simulink model "SF007A_SysFricLrng"  (R2013b)
settings: Solver=FixedStepDiscrete  SolverMode=SingleTasking  StartTime=0.0  StopTime=1  FixedStep=0.002  RelTol=1e-3
PostLoadFcn:
  | , if any(exist('dsrtsu_mdlpostloadfcn', 'file') == [2, 3, 6]), try dsrtsu_mdlpostloadfcn('Execute', bdroot); catch fprintf('Error in PostLoadFcn (dsrtsu_mdlpostloadfcn) for model "%s":\n %s\n', bdroot, lasterr); end, end,
undefined symbols (not defined in the file): ARCHGLBPRM_100MILLISEC_SEC_F32, ARCHGLBPRM_10MILLISEC_SEC_F32, ARCHGLBPRM_180OVERPI_ULS_F32, CONV100MICROSECTOSEC_ULS_F32, FLTINJ_SYSFRICLRNG_SYSFRICOFFS, FricLrngData, HiFricNtc, HWPTNUM_CNT_U08, HWPTNUMSUB1_CNT_U08, HWVELDECDIR_ULS_U08, HWVELINCDIR_ULS_U08, IDXCALCNSCAGFAC_ULS_U08, IDXSELN1_ULS_U08, IDXSELN2_ULS_U08, IDXSELN3_ULS_U08, LRNGENASCAFAC_MILLISEC_U32, NtcSts1, SCAGFACQUARTER_CNT_F32, SCAGFACTEN_CNT_U16, SECIDXSELN_ULS_U08, SysFricLrngBasLineEolFric, SysFricLrngBasLineFric, SysFricLrngBasLineHys, SysFricLrngBasLineRngCntr, SysFricLrngEolFricDifScagFac, SysFricLrngFricChgWght, SysFricLrngFricDiagcThd, SysFricLrngFricDiagcTiThd, SysFricLrngFricHysHwAgPt, SysFricLrngGain, SysFricLrngHwPosnAuthyThd, SysFricLrngHwVelConstrLim, SysFricLrngHwVelHiLim, SysFricLrngHwVelLoLim, SysFricLrngIgnCycFricChgLim, SysFricLrngLatAHiLim, SysFricLrngLatALoLim, SysFricLrngMaskVehSpd, SysFricLrngOperMod1, SysFricLrngRngCntrThd, SysFricLrngThd, SysFricLrngTHiLim, SysFricLrngTLoLim, SysFricLrngVehSpd, SYSFRICOFFSLIM_HWNWTMTR_F32, VEHSPDPTNUM1_ULS_U08, VEHSPDPTNUM2_ULS_U08
libraries: Fil x19, simulink x17, NxtrLim x10, NxtrAbslt x3, NxtrNvM x2, FixdToFloat x2, FloatToFixd x1, LnrIntrpn x1
(part 4 of 7)

== system SF007A_SysFricLrng/SysFricLrng/SysFricLrngPer1/RunningAndCalibrationModes/FricLearning/Gate Calculation ==
  SelHwAg : Inport
  IC : Inport  Port=2
  Add1 : Sum
  Constant2 : Constant  Value=HWPTNUMSUB1_CNT_U08
  Constant3 : Constant  Value=SysFricLrngFricHysHwAgPt
  Constant4 : Constant  OutDataTypeStr=uint8
      settings: AttributesFormatString=%<OutDataTypeStr>
  CopyRight2 : Subsystem  Description=|  mask(Copyright Information){none=on}
      | Copyright info block.                                               
      |                                                                     
      | Place copyright information at the top of every subsystem in design.
      mask prompts: none "No parameters"
      mask help: Place copyright information at the top of every subsystem in design.
      mask Display:
      | NxtrConf = 'Nexteer Confidential';
      | 
      | sys = bdroot; %handle for the current model ("system")
      | first = get_param(sys,'Created');
      | first = first(end-3:end);  %year is last four digits
      | 
      | last = get_param(sys,'LastModifiedDate');
      | if isempty(last)
      |     last = datestr(now,'yyyy');
      | else
      |     last = last(end-3:end);
      | end
      | 
      | if strcmp(first,last)
      |     fprintf('%s -- Copyright %s Nexteer',NxtrConf,first)
      | else
      |     fprintf('%s -- %s%s- %s Nexteer',NxtrConf,char(169),first,last)
      | end
  Logical Operator : Logic  AllPortsSameDT=off  OutDataTypeStr=boolean
  Logical Operator1 : Logic  Operator=OR  AllPortsSameDT=off  OutDataTypeStr=boolean
  Relational Operator : RelationalOperator  Operator=<  OutDataTypeStr=boolean
  Relational Operator1 : RelationalOperator  Operator=<  OutDataTypeStr=boolean
  Relational Operator2 : RelationalOperator  OutDataTypeStr=boolean
  Selector : Selector  IndexOptions=Index vector (port)  Indices=[1 3]  OutputSizes=1
  Selector1 : Selector  IndexOptions=Index vector (port)  Indices=[1 3]  OutputSizes=1
  While Iterator : WhileIterator  MaxIters=-1  ShowIterationPort=on
  Gate : Outport
  wires:
  IC/1 -> While Iterator/2
  Constant3/1 -> Selector/1, Selector1/1
  Constant2/1 -> Relational Operator/2
  Relational Operator/1 -> Logical Operator/1
  Add1/1 -> Selector1/2
  Constant4/1 -> Add1/2
  Logical Operator1/1 -> Logical Operator/2
  Logical Operator/1 -> While Iterator/1
  SelHwAg/1 -> [SelHwAg]
  [SelHwAg] -> Relational Operator1/1
  Selector/1 -> Relational Operator1/2
  Relational Operator1/1 -> Logical Operator1/1
  Selector1/1 -> Relational Operator2/2
  [SelHwAg] -> Relational Operator2/1
  Relational Operator2/1 -> Logical Operator1/2
  While Iterator/1 -> Gate/1, Relational Operator/1, Selector/2, Add1/1

== system SF007A_SysFricLrng/SysFricLrng/SysFricLrngPer1/RunningAndCalibrationModes/FricLearning/Indices Calculation ==
  note: Code: (Zero Based Index)                       ||   Model (One Based Index)
      | -----------------------------------------------------||----------------------------------------------------
      | VSIdx | OffsInc | OffsDec|Offs(0)|Offs(1) ||VSIdx | OffsInc | OffsDec|Offs(0)|Offs(1)
      | -----------------------------------------------------------------------------------------------------------
      |      0    |    0      |  1          |  0       |    1      ||   1      |   1         |  2         | 1      |   2
      |      1    |    2      |  3          |  2       |    3      ||   2      |   3         |  4         | 3      |   4
      |      2    |    4      |  5          |  4       |    5      ||   3      |   5         |  6         | 5      |   6
      |      3    |    6      |  7          |  6       |    7      ||   4      |   7         |  8         | 7      |   8
  note: Note: Mapping of values between Zero Based and one based Index
  HwVelDir : Inport
  VehSpdIdx : Inport  Port=2
  Add1 : Sum  Inputs=+-
  Add2 : Sum
  Add3 : Sum  Inputs=+-
  Constant1 : Constant  OutDataTypeStr=uint8
      settings: AttributesFormatString=%<OutDataTypeStr>
  Constant2 : Constant  Value=IDXCALCNSCAGFAC_ULS_U08
  Constant3 : Constant  OutDataTypeStr=uint8
      settings: AttributesFormatString=%<OutDataTypeStr>
  CopyRight2 : Subsystem  Description=|  mask(Copyright Information){none=on}
      | Copyright info block.                                               
      |                                                                     
      | Place copyright information at the top of every subsystem in design.
      mask prompts: none "No parameters"
      mask help: Place copyright information at the top of every subsystem in design.
      mask Display:
      | NxtrConf = 'Nexteer Confidential';
      | 
      | sys = bdroot; %handle for the current model ("system")
      | first = get_param(sys,'Created');
      | first = first(end-3:end);  %year is last four digits
      | 
      | last = get_param(sys,'LastModifiedDate');
      | if isempty(last)
      |     last = datestr(now,'yyyy');
      | else
      |     last = last(end-3:end);
      | end
      | 
      | if strcmp(first,last)
      |     fprintf('%s -- Copyright %s Nexteer',NxtrConf,first)
      | else
      |     fprintf('%s -- %s%s- %s Nexteer',NxtrConf,char(169),first,last)
      | end
  Product : Product
  DeltaIdxOffsInc : Outport
  DeltaIdxOffs : Outport  Port=2
  DeltaIdxOffsDec : Outport  Port=3
  wires:
  Product/1 -> DeltaIdxOffsDec/1, Add3/1, Add2/2
  HwVelDir/1 -> Add2/1
  Constant2/1 -> Product/2
  VehSpdIdx/1 -> Product/1
  Add3/1 -> DeltaIdxOffsInc/1
  Constant3/1 -> Add3/2
  Add2/1 -> Add1/1
  Add1/1 -> DeltaIdxOffs/1
  Constant1/1 -> Add1/2

== stateflow chart SF007A_SysFricLrng/SysFricLrng/SysFricLrngPer1/RunningAndCalibrationModes/FricLearning/Calculate Average Friction/NTC PASS /SetNtcSts/SetNtcSts/ISO Fault Debounce Design ==
  note: NTCSTS_PASSD           (0)
      | NTCSTS_FAILD             (1)
      | NTCSTS_PREPASSD   (2)
      | NTCSTS_PREFAILD     (3)
      |
      | SIGQLFR_NORES        (0)
      | SIGQLFR_PASSD         (1)
      | SIGQLFR_FAILD           (2)
  note: Pass Loop
  note: Fail Loop
  note: 
  (default) -> (junction 89)
  (junction 89) -> (junction 95) [order 1] : [NtcSts ==3]
  (junction 89) -> (junction 93) [order 2] : [NtcSts ==2]
  (junction 89) -> (junction 141) [order 3] : [NtcSts ==1]
      | { ErrAcc = 32767;
      | Qualifier =2;
      |  }
  (junction 89) -> (junction 141) [order 4] : [NtcSts ==0]
      | { ErrAcc = -32768;
      | Qualifier=1;
      | }
  (junction 95) -> (junction 103) [order 2]
  (junction 95) -> (junction 111) [order 1] : [ErrAcc <=0]
      | {ErrAcc = DebStep;}
  (junction 93) -> (junction 123) [order 2] : {
      | ErrAcc = ErrAcc - DebStep;
      | }
  (junction 93) -> (junction 123) [order 1] : [(ErrAcc - DebStep) <= -32768]
      | { ErrAcc = -32768;
      | Qualifier=1;
      | }
  (junction 103) -> (junction 111) [order 1] : [(ErrAcc + DebStep) <32767]
      | {ErrAcc = ErrAcc + DebStep;}
  (junction 103) -> (junction 111) [order 2] : {ErrAcc = 32767;
      | Qualifier =2;}
  (junction 123) -> (junction 141)
  (junction 111) -> (junction 141)
  (junction 141) -> (junction 159) [order 2] : {ErrAcc = 0;
      | Qualifier =0;
      | }
  (junction 141) -> (junction 159) [order 1] : [SvcClr ==0]
  data: NtcSts input Enum: NtcSts1; Qualifier output uint8; DebStep input uint16; ErrAcc local single; SvcClr input

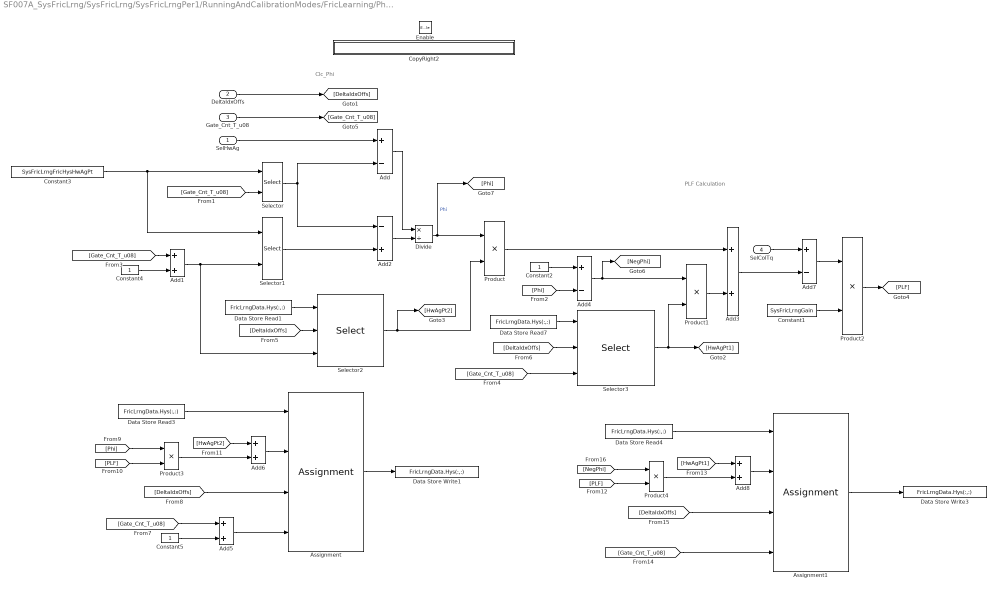
== system SF007A_SysFricLrng/SysFricLrng/SysFricLrngPer1/RunningAndCalibrationModes/FricLearning/Phi Calculation ==
  note: Clc_Phi
  note: PLF Calculation
  SelHwAg : Inport
  DeltaIdxOffs : Inport  Port=2
  Gate_Cnt_T_u08 : Inport  Port=3
  SelColTq : Inport  Port=4
  Enable : EnablePort
  Add : Sum  Inputs=+-
  Add{1,3,5..6,8} (5 alike) : Sum
  Add2 : Sum  Inputs=-+
  Add4 : Sum  Inputs=+-
  Add7 : Sum  Inputs=+-
  Assignment : Assignment  NumberOfDimensions=2  IndexOptions=Index vector (port),Index vector (port)  Indices=1,1  OutputSizes=1,1
  Assignment1 : Assignment  NumberOfDimensions=2  IndexOptions=Index vector (port),Index vector (port)  Indices=1,1  OutputSizes=1,1
  Constant1 : Constant  Value=SysFricLrngGain
  Constant2 : Constant  OutDataTypeStr=single
      settings: AttributesFormatString=%<OutDataTypeStr>
  Constant3 : Constant  Value=SysFricLrngFricHysHwAgPt
  Constant4 : Constant  OutDataTypeStr=uint16
      settings: AttributesFormatString=%<OutDataTypeStr>
  Constant5 : Constant  OutDataTypeStr=uint16
      settings: AttributesFormatString=%<OutDataTypeStr>
  CopyRight2 : Subsystem  Description=|  mask(Copyright Information){none=on}
      | Copyright info block.                                               
      |                                                                     
      | Place copyright information at the top of every subsystem in design.
      mask prompts: none "No parameters"
      mask help: Place copyright information at the top of every subsystem in design.
      mask Display:
      | NxtrConf = 'Nexteer Confidential';
      | 
      | sys = bdroot; %handle for the current model ("system")
      | first = get_param(sys,'Created');
      | first = first(end-3:end);  %year is last four digits
      | 
      | last = get_param(sys,'LastModifiedDate');
      | if isempty(last)
      |     last = datestr(now,'yyyy');
      | else
      |     last = last(end-3:end);
      | end
      | 
      | if strcmp(first,last)
      |     fprintf('%s -- Copyright %s Nexteer',NxtrConf,first)
      | else
      |     fprintf('%s -- %s%s- %s Nexteer',NxtrConf,char(169),first,last)
      | end
  Data Store Read{1,3..4,7} (4 alike) : DataStoreRead  Priority=1  DataStoreName=FricLrngData  DataStoreElements=FricLrngData.Hys(:,:)
      settings: AttributesFormatString=Priority: %<Priority>
  Data Store Write1 : DataStoreWrite  Priority=2  DataStoreName=FricLrngData  DataStoreElements=FricLrngData.Hys(:,:)
      settings: AttributesFormatString=Priority: %<Priority>
  Data Store Write3 : DataStoreWrite  Priority=2  DataStoreName=FricLrngData  DataStoreElements=FricLrngData.Hys(:,:)
      settings: AttributesFormatString=Priority: %<Priority>
  Divide : Product  Inputs=*/
  Product{,1..4} (5 alike) : Product
  Selector : Selector  IndexOptions=Index vector (port)  Indices=[1 3]  OutputSizes=1
  Selector1 : Selector  IndexOptions=Index vector (port)  Indices=[1 3]  OutputSizes=1
  Selector2 : Selector  NumberOfDimensions=2  IndexOptions=Index vector (port),Index vector (port)  Indices=[1 3],1  OutputSizes=1,1
  Selector3 : Selector  NumberOfDimensions=2  IndexOptions=Index vector (port),Index vector (port)  Indices=[1 3],1  OutputSizes=1,1
  wires:
  Constant3/1 -> Selector1/1, Selector/1
  [Gate_Cnt_T_u08] -> Selector/2
  SelHwAg/1 -> Add/1
  Selector/1 -> Add/2, Add2/1
  Add/1 -> Divide/1
  Divide/1 -> Product/1, [Phi]  "Phi"
  Add1/1 -> Selector1/2, Selector2/3
  [Gate_Cnt_T_u08] -> Add1/1
  Constant4/1 -> Add1/2
  Selector1/1 -> Add2/2
  Add2/1 -> Divide/2
  Data Store Read1/1 -> Selector2/1
  [DeltaIdxOffs] -> Selector2/2
  Selector2/1 -> Product/2, [HwAgPt2]
  Product/1 -> Add3/1
  Constant2/1 -> Add4/1
  [Phi] -> Add4/2
  Data Store Read7/1 -> Selector3/1
  [Gate_Cnt_T_u08] -> Selector3/3
  DeltaIdxOffs/1 -> [DeltaIdxOffs]
  [DeltaIdxOffs] -> Selector3/2
  Add4/1 -> Product1/1, [NegPhi]
  Selector3/1 -> Product1/2, [HwAgPt1]
  Product1/1 -> Add3/2
  Constant1/1 -> Product2/2
  [Gate_Cnt_T_u08] -> Add5/1
  Constant5/1 -> Add5/2
  [DeltaIdxOffs] -> Assignment/3
  Add5/1 -> Assignment/4
  Assignment/1 -> Data Store Write1/1
  Data Store Read3/1 -> Assignment/1
  Product2/1 -> [PLF]
  Product3/1 -> Add6/2
  Add6/1 -> Assignment/2
  [Phi] -> Product3/1
  [PLF] -> Product3/2
  [HwAgPt2] -> Add6/1
  [DeltaIdxOffs] -> Assignment1/3
  Assignment1/1 -> Data Store Write3/1
  Data Store Read4/1 -> Assignment1/1
  Product4/1 -> Add8/2
  Add8/1 -> Assignment1/2
  [NegPhi] -> Product4/1
  [PLF] -> Product4/2
  [HwAgPt1] -> Add8/1
  [Gate_Cnt_T_u08] -> Assignment1/4
  Add3/1 -> Add7/2
  SelColTq/1 -> Add7/1
  Add7/1 -> Product2/1
  Gate_Cnt_T_u08/1 -> [Gate_Cnt_T_u08]

== system SF007A_SysFricLrng/SysFricLrng/SysFricLrngPer1/RunningAndCalibrationModes/FricLearning/Range Counter Manager ==
  note: Added ONE here to make the entry condition for phi calculation
      | check for three times i.e., gate = 0,1,2 as per code.(Line: 1725)
      | Here It compares for Gate = 1,2,3 as Gate starts from 1.
      | This is only for MATLAB simulation purpose
  "DeltaIdxOffs " : Inport
  DeltaIdxOffsInc : Inport  Port=2
  DeltaIdxOffsDec : Inport  Port=3
  Gate_Cnt_T_u08 : Inport  Port=4
  Add : Sum
  Constant1 : Constant  Value=0  OutDataTypeStr=boolean
      settings: AttributesFormatString=%<OutDataTypeStr>
  Constant2 : Constant  Value=HWPTNUMSUB1_CNT_U08
  Constant3 : Constant  Value=HWPTNUMSUB1_CNT_U08
  Constant5 : Constant  OutDataTypeStr=uint16
      settings: AttributesFormatString=%<OutDataTypeStr>
  CopyRight2 : Subsystem  Description=|  mask(Copyright Information){none=on}
      | Copyright info block.                                               
      |                                                                     
      | Place copyright information at the top of every subsystem in design.
      mask prompts: none "No parameters"
      mask help: Place copyright information at the top of every subsystem in design.
      mask Display:
      | NxtrConf = 'Nexteer Confidential';
      | 
      | sys = bdroot; %handle for the current model ("system")
      | first = get_param(sys,'Created');
      | first = first(end-3:end);  %year is last four digits
      | 
      | last = get_param(sys,'LastModifiedDate');
      | if isempty(last)
      |     last = datestr(now,'yyyy');
      | else
      |     last = last(end-3:end);
      | end
      | 
      | if strcmp(first,last)
      |     fprintf('%s -- Copyright %s Nexteer',NxtrConf,first)
      | else
      |     fprintf('%s -- %s%s- %s Nexteer',NxtrConf,char(169),first,last)
      | end
  Data Store Memory12 : DataStoreMemory  Description=Local Data Store Memory  DataStoreName=RngCntrThdExcdd_Cnt_T_lgc  ReadBeforeWriteMsg=warning  WriteAfterWriteMsg=warning  WriteAfterReadMsg=warning  OutDataTypeStr=boolean
      settings: AttributesFormatString=%<Description>
  Data Store Read6 : DataStoreRead  Priority=1  DataStoreName=RngCntrThdExcdd_Cnt_T_lgc
      settings: AttributesFormatString=Priority:%<Priority>
  Data Store Write1 : DataStoreWrite  Priority=1  DataStoreName=RngCntrThdExcdd_Cnt_T_lgc
      settings: AttributesFormatString=Priority:%<Priority>
  Range Counter Control : Subsystem  TreatAsAtomicUnit=on
  Range Counter Control1 : Subsystem  TreatAsAtomicUnit=on
  Range Counter Threshold Calculation : Subsystem  Priority=1  TreatAsAtomicUnit=on
  Relational Operator : RelationalOperator  Operator=<  OutDataTypeStr=boolean
  wires:
  "DeltaIdxOffs "/1 -> Range Counter Threshold Calculation/2(DeltaIdxOffs), Range Counter Control/2(DeltaIdxOffs)
  Constant1/1 -> Data Store Write1/1
  Gate_Cnt_T_u08/1 -> Relational Operator/1, Range Counter Control/1(Gate_Cnt_T_u08)
  Relational Operator/1 -> Range Counter Control/Enable
  Data Store Read6/1 -> Range Counter Control1/Enable
  DeltaIdxOffsInc/1 -> Range Counter Control1/1(DeltaIdxOffsInc)
  DeltaIdxOffsDec/1 -> Range Counter Control1/2(DeltaIdxOffsDec)
  Constant3/1 -> Range Counter Threshold Calculation/1(HWPTNUMSUB1_CNT_U08)
  Constant5/1 -> Add/2
  Add/1 -> Relational Operator/2
  Constant2/1 -> Add/1

== system SF007A_SysFricLrng/SysFricLrng/SysFricLrngPer1/RunningAndCalibrationModes/Hold Last value/CopyRight2 ==

== system SF007A_SysFricLrng/SysFricLrng/SysFricLrngPer1/RunningAndCalibrationModes/LearningConstraint/ColTqconstraint ==
  note: Note: Comment edited to ensure clarity and prevent confusion ; No code change required
  note: This comment is defined here to differentiate between design and its requirement. Since other constraint
      |  blocks use a size of 12 ,we need to  use same buffer of 12 to avoid phase shifting relative to other signals
      |  that are also buffering.
  ColTq : Inport
  ColTqAryCalcn : Subsystem
  CopyRight2 : Subsystem  Description=|  mask(Copyright Information){none=on}
      | Copyright info block.                                               
      |                                                                     
      | Place copyright information at the top of every subsystem in design.
      mask prompts: none "No parameters"
      mask help: Place copyright information at the top of every subsystem in design.
      mask Display:
      | NxtrConf = 'Nexteer Confidential';
      | 
      | sys = bdroot; %handle for the current model ("system")
      | first = get_param(sys,'Created');
      | first = first(end-3:end);  %year is last four digits
      | 
      | last = get_param(sys,'LastModifiedDate');
      | if isempty(last)
      |     last = datestr(now,'yyyy');
      | else
      |     last = last(end-3:end);
      | end
      | 
      | if strcmp(first,last)
      |     fprintf('%s -- Copyright %s Nexteer',NxtrConf,first)
      | else
      |     fprintf('%s -- %s%s- %s Nexteer',NxtrConf,char(169),first,last)
      | end
  SelColTq : Outport
  wires:
  ColTq/1 -> ColTqAryCalcn/1(ColTq)
  ColTqAryCalcn/1(SelColTq) -> SelColTq/1

== system SF007A_SysFricLrng/SysFricLrng/SysFricLrngPer1/RunningAndCalibrationModes/LearningConstraint/CopyRight2 ==

== system SF007A_SysFricLrng/SysFricLrng/SysFricLrngPer1/RunningAndCalibrationModes/LearningConstraint/Existing System Time ==
  Action Port : ActionPort  ActionType=else
  CopyRight2 : Subsystem  Description=|  mask(Copyright Information){none=on}
      | Copyright info block.                                               
      |                                                                     
      | Place copyright information at the top of every subsystem in design.
      mask prompts: none "No parameters"
      mask help: Place copyright information at the top of every subsystem in design.
      mask Display:
      | NxtrConf = 'Nexteer Confidential';
      | 
      | sys = bdroot; %handle for the current model ("system")
      | first = get_param(sys,'Created');
      | first = first(end-3:end);  %year is last four digits
      | 
      | last = get_param(sys,'LastModifiedDate');
      | if isempty(last)
      |     last = datestr(now,'yyyy');
      | else
      |     last = last(end-3:end);
      | end
      | 
      | if strcmp(first,last)
      |     fprintf('%s -- Copyright %s Nexteer',NxtrConf,first)
      | else
      |     fprintf('%s -- %s%s- %s Nexteer',NxtrConf,char(169),first,last)
      | end
  Data Store Read : DataStoreRead  DataStoreName=RefTmrLrngConstr
  RefTmrLrngConstr : Outport
  wires:
  Data Store Read/1 -> RefTmrLrngConstr/1

== system SF007A_SysFricLrng/SysFricLrng/SysFricLrngPer1/RunningAndCalibrationModes/LearningConstraint/Get System Time ==
  Action Port : ActionPort  ActionType=then
  CopyRight2 : Subsystem  Description=|  mask(Copyright Information){none=on}
      | Copyright info block.                                               
      |                                                                     
      | Place copyright information at the top of every subsystem in design.
      mask prompts: none "No parameters"
      mask help: Place copyright information at the top of every subsystem in design.
      mask Display:
      | NxtrConf = 'Nexteer Confidential';
      | 
      | sys = bdroot; %handle for the current model ("system")
      | first = get_param(sys,'Created');
      | first = first(end-3:end);  %year is last four digits
      | 
      | last = get_param(sys,'LastModifiedDate');
      | if isempty(last)
      |     last = datestr(now,'yyyy');
      | else
      |     last = last(end-3:end);
      | end
      | 
      | if strcmp(first,last)
      |     fprintf('%s -- Copyright %s Nexteer',NxtrConf,first)
      | else
      |     fprintf('%s -- %s%s- %s Nexteer',NxtrConf,char(169),first,last)
      | end
  Data Store Write : DataStoreWrite  DataStoreName=RefTmrLrngConstr
  GetRefTmr100MicroSec32bit : Subsystem
  RefTmrLrngConstr : Outport
  wires:
  GetRefTmr100MicroSec32bit/1(RefTmr) -> Data Store Write/1, RefTmrLrngConstr/1

== system SF007A_SysFricLrng/SysFricLrng/SysFricLrngPer1/RunningAndCalibrationModes/LearningConstraint/GetTiSpan100MicroSec32bit ==
  note: Subtract original reference time
  note: seconds
  note: microseconds
  note: counts
  note: Wrap-to-zero
  note: 1 count = 100 uSec
  note: Get current system time
  note: GetTiSpan100MicroSec32bit
  note: Created Aug 18, 2015
      | Modified Oct 21, 2015
      | Modified Oct 30, 2015
      | Kevin Derry
  RefTmr : Inport
  CopyRight2 : Subsystem  Description=|  mask(Copyright Information){none=on}
      | Copyright info block.                                               
      |                                                                     
      | Place copyright information at the top of every subsystem in design.
      mask prompts: none "No parameters"
      mask help: Place copyright information at the top of every subsystem in design.
      mask Display:
      | NxtrConf = 'Nexteer Confidential';
      | 
      | sys = bdroot; %handle for the current model ("system")
      | first = get_param(sys,'Created');
      | if(isempty(first))
      |     first = datestr(now,'yyyy');
      | else
      |     first = first(end-3:end);  %year is last four digits
      | end
      | 
      | last = get_param(sys,'LastModifiedDate');
      | if isempty(last)
      |     last = datestr(now,'yyyy');
      | else
      |     last = last(end-3:end);
      | end
      | 
      | if strcmp(first,last)
      |     fprintf('%s -- Copyright %s Nexteer',NxtrConf,first)
      | else
      |     fprintf('%s -- %s%s- %s Nexteer',NxtrConf,char(169),first,last)
      | end
  Count per uSec : Constant  Value=0.01
  Data Store Read1 : DataStoreRead  DataStoreName=SimnTi
  Data Type Conversion2 : DataTypeConversion  OutDataTypeStr=uint32
  Divide1 : Product  Inputs=**
  Divide2 : Product  Inputs=*/
  If : If  NumInputs=2  IfExpression=u1 >= u2
  Max Counts : Constant  Value=2^32-1
  Merge : Merge
  No wrapping : Subsystem  TreatAsAtomicUnit=on
  Product2 : Product
  Product3 : Product
  Rounding : Rounding
  Subtract3 : Sum  Inputs=+-
  Wrapping : Subsystem  TreatAsAtomicUnit=on
  uSec per Sec : Constant  Value=1000000
  TiSpan : Outport
  wires:
  Wrapping/1(Out1) -> Merge/2
  No wrapping/1(Out1) -> Merge/1
  If/2 -> Wrapping/Action
  If/1 -> No wrapping/Action
  Product3/1 -> Subtract3/2
  Subtract3/1 -> Data Type Conversion2/1
  Rounding/1 -> Product3/1
  Divide2/1 -> Rounding/1
  Max Counts/1 -> Divide2/2, Product3/2
  Divide1/1 -> Divide2/1, Subtract3/1
  Product2/1 -> Divide1/1
  Data Store Read1/1 -> Product2/1
  Count per uSec/1 -> Divide1/2
  uSec per Sec/1 -> Product2/2
  Merge/1 -> TiSpan/1
  RefTmr/1 -> If/2, No wrapping/2(ref), Wrapping/2(ref)
  Data Type Conversion2/1 -> If/1, No wrapping/1(new), Wrapping/1(new)

== system SF007A_SysFricLrng/SysFricLrng/SysFricLrngPer1/RunningAndCalibrationModes/LearningConstraint/HwAngConstraint ==
  note: No of ouputs = FricLrn_d_BufferDepth i.e., 12
  note: Create a buffer of 12 Hw angle values.
      | All 12 values must lie between the min and max values of calibration table.
      | Otuput a Hw angle value from the middle of buffer and a flag to indicate whether all buffered points met the requirment.
  HwAg : Inport
  Constant : Constant  Value=SysFricLrngFricHysHwAgPt
  CopyRight2 : Subsystem  Description=|  mask(Copyright Information){none=on}
      | Copyright info block.                                               
      |                                                                     
      | Place copyright information at the top of every subsystem in design.
      mask prompts: none "No parameters"
      mask help: Place copyright information at the top of every subsystem in design.
      mask Display:
      | NxtrConf = 'Nexteer Confidential';
      | 
      | sys = bdroot; %handle for the current model ("system")
      | first = get_param(sys,'Created');
      | first = first(end-3:end);  %year is last four digits
      | 
      | last = get_param(sys,'LastModifiedDate');
      | if isempty(last)
      |     last = datestr(now,'yyyy');
      | else
      |     last = last(end-3:end);
      | end
      | 
      | if strcmp(first,last)
      |     fprintf('%s -- Copyright %s Nexteer',NxtrConf,first)
      | else
      |     fprintf('%s -- %s%s- %s Nexteer',NxtrConf,char(169),first,last)
      | end
  Data Store Read1 : DataStoreRead  DataStoreName=HwAgBuf
  Demux : Demux  Outputs=12
  Handwheel Angle Buffer : Subsystem
  Interval Test Dynamic : simulink/Logic and Bit Operations/Interval Test Dynamic  IntervalClosedRight=on  IntervalClosedLeft=on  OutDataTypeStr=boolean
  Logical Operator : Logic  Inputs=12  AllPortsSameDT=off  OutDataTypeStr=boolean
  Selector : Selector  InputPortWidth=4  IndexOptions=Index vector (dialog)  Indices=[1]  OutputSizes=1
  Selector1 : Selector  InputPortWidth=4  IndexOptions=Index vector (dialog)  Indices=4  OutputSizes=1
  HwAgOk : Outport
  SelHwAg : Outport  Port=2
  wires:
  Selector1/1 -> Interval Test Dynamic/1
  Constant/1 -> Selector1/1, Selector/1
  Selector/1 -> Interval Test Dynamic/3
  Interval Test Dynamic/1 -> Demux/1
  Demux/1 -> Logical Operator/1
  Demux/2 -> Logical Operator/2
  Demux/3 -> Logical Operator/3
  Demux/4 -> Logical Operator/4
  Demux/5 -> Logical Operator/5
  Demux/6 -> Logical Operator/6
  Demux/7 -> Logical Operator/7
  Demux/8 -> Logical Operator/8
  Logical Operator/1 -> HwAgOk/1
  Demux/9 -> Logical Operator/9
  Demux/10 -> Logical Operator/10
  Demux/11 -> Logical Operator/11
  Demux/12 -> Logical Operator/12
  HwAg/1 -> Handwheel Angle Buffer/1(HwAg)
  Handwheel Angle Buffer/1(SelHwAg) -> SelHwAg/1
  Data Store Read1/1 -> Interval Test Dynamic/2

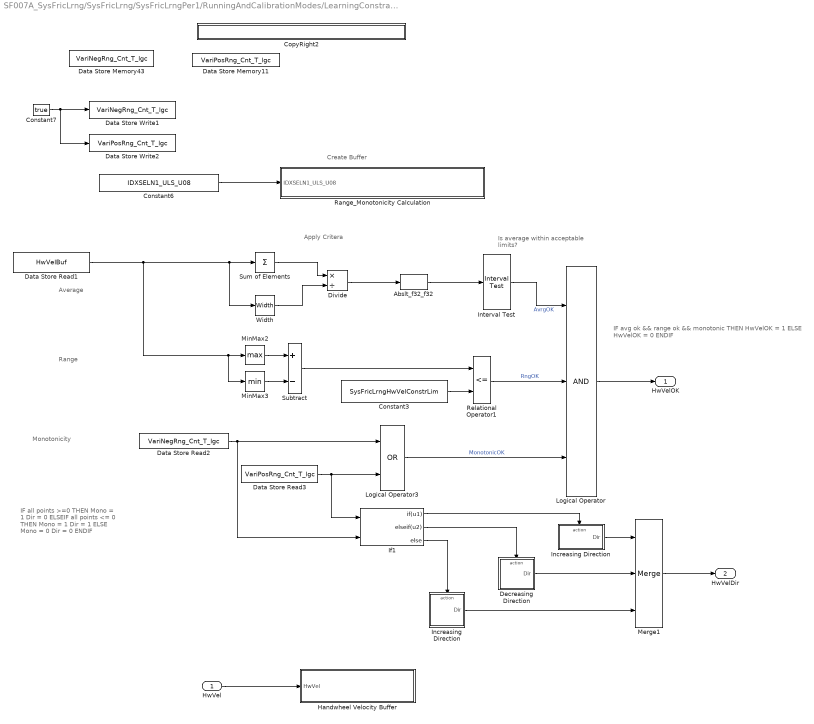
== system SF007A_SysFricLrng/SysFricLrng/SysFricLrngPer1/RunningAndCalibrationModes/LearningConstraint/HwVelConstraint ==
  note: Create Buffer
  note: IF all points >=0 THEN
      |    Mono = 1
      |    Dir     = 0
      | ELSEIF all points <= 0 THEN
      |    Mono = 1
      |    Dir     = 1
      | ELSE
      |    Mono = 0
      |    Dir     = 0
      | ENDIF
  note: IF avg ok && range ok && monotonic THEN
      |    HwVelOK = 1
      | ELSE
      |    HwVelOK = 0
      | ENDIF
  note: Is average within acceptable limits?
  note: Apply Critera
  note: Average
  note: Range
  note: Monotonicity
  HwVel : Inport
  Abslt_f32_f32 : NxtrAbslt/Abslt_f32_f32  SFunctionSpec=single y1 = Abslt_f32_f32(single u1)
      settings: AttributesFormatString=%<Name>
  Constant3 : Constant  Value=SysFricLrngHwVelConstrLim
  Constant6 : Constant  Value=IDXSELN1_ULS_U08
  Constant7 : Constant  Value=true  OutDataTypeStr=boolean
      settings: AttributesFormatString=%<OutDataTypeStr>
  CopyRight2 : Subsystem  Description=|  mask(Copyright Information){none=on}
      | Copyright info block.                                               
      |                                                                     
      | Place copyright information at the top of every subsystem in design.
      mask prompts: none "No parameters"
      mask help: Place copyright information at the top of every subsystem in design.
      mask Display:
      | NxtrConf = 'Nexteer Confidential';
      | 
      | sys = bdroot; %handle for the current model ("system")
      | first = get_param(sys,'Created');
      | first = first(end-3:end);  %year is last four digits
      | 
      | last = get_param(sys,'LastModifiedDate');
      | if isempty(last)
      |     last = datestr(now,'yyyy');
      | else
      |     last = last(end-3:end);
      | end
      | 
      | if strcmp(first,last)
      |     fprintf('%s -- Copyright %s Nexteer',NxtrConf,first)
      | else
      |     fprintf('%s -- %s%s- %s Nexteer',NxtrConf,char(169),first,last)
      | end
  Data Store Memory11 : DataStoreMemory  Description=Local Data Store Memory  DataStoreName=VariPosRng_Cnt_T_lgc  ReadBeforeWriteMsg=warning  WriteAfterWriteMsg=warning  WriteAfterReadMsg=warning  OutDataTypeStr=boolean
      settings: AttributesFormatString=%<Description>
  Data Store Memory43 : DataStoreMemory  Description=Local Data Store Memory  DataStoreName=VariNegRng_Cnt_T_lgc  ReadBeforeWriteMsg=warning  WriteAfterWriteMsg=warning  WriteAfterReadMsg=warning  OutDataTypeStr=boolean
      settings: AttributesFormatString=%<Description>
  Data Store Read1 : DataStoreRead  DataStoreName=HwVelBuf
  Data Store Read2 : DataStoreRead  Priority=2  DataStoreName=VariNegRng_Cnt_T_lgc
      settings: AttributesFormatString=Priority:%<Priority>
  Data Store Read3 : DataStoreRead  Priority=2  DataStoreName=VariPosRng_Cnt_T_lgc
      settings: AttributesFormatString=Priority:%<Priority>
  Data Store Write1 : DataStoreWrite  Priority=1  DataStoreName=VariNegRng_Cnt_T_lgc
      settings: AttributesFormatString=Priority:%<Priority>
  Data Store Write2 : DataStoreWrite  Priority=1  DataStoreName=VariPosRng_Cnt_T_lgc
      settings: AttributesFormatString=Priority:%<Priority>
  Decreasing Direction : Subsystem  TreatAsAtomicUnit=on
  Divide : Product  Inputs=*/
  Handwheel Velocity Buffer : Subsystem
  If1 : If  NumInputs=2  IfExpression=u1  ElseIfExpressions=u2
  Increasing Direction : Subsystem  TreatAsAtomicUnit=on
  Increasing Direction : Subsystem  TreatAsAtomicUnit=on
  Interval Test : simulink/Logic and Bit Operations/Interval Test  IntervalClosedRight=on  uplimit=SysFricLrngHwVelHiLim  IntervalClosedLeft=on  lowlimit=SysFricLrngHwVelLoLim  OutDataTypeStr=boolean
  Logical Operator : Logic  Inputs=3  AllPortsSameDT=off  OutDataTypeStr=boolean
  Logical Operator3 : Logic  Operator=OR  AllPortsSameDT=off  OutDataTypeStr=boolean
  Merge1 : Merge  Inputs=3
  MinMax2 : MinMax  Function=max
  MinMax3 : MinMax
  Range_Monotonicity Calculation : Subsystem  Priority=1  TreatAsAtomicUnit=on
      settings: AttributesFormatString=Priority:%<Priority>
  Relational Operator1 : RelationalOperator  Operator=<=  OutDataTypeStr=boolean
  Subtract : Sum  Inputs=+-
  Sum of Elements : Sum  Inputs=+
  Width : Width  DataType=single
  HwVelOK : Outport
  HwVelDir : Outport  Port=2
  wires:
  MinMax2/1 -> Subtract/1
  MinMax3/1 -> Subtract/2
  Subtract/1 -> Relational Operator1/1
  Relational Operator1/1 -> Logical Operator/2  "RngOK"
  Divide/1 -> Abslt_f32_f32/1
  Interval Test/1 -> Logical Operator/1  "AvrgOK"
  Constant3/1 -> Relational Operator1/2
  Abslt_f32_f32/1 -> Interval Test/1
  Logical Operator/1 -> HwVelOK/1
  Logical Operator3/1 -> Logical Operator/3  "MonotonicOK"
  If1/1 -> Increasing Direction/Action
  If1/2 -> Decreasing Direction/Action
  If1/3 -> Increasing Direction/Action
  Increasing Direction/1(Dir) -> Merge1/1
  Decreasing Direction/1(Dir) -> Merge1/2
  Increasing Direction/1(Dir) -> Merge1/3
  Merge1/1 -> HwVelDir/1
  HwVel/1 -> Handwheel Velocity Buffer/1(HwVel)
  Sum of Elements/1 -> Divide/1
  Data Store Read1/1 -> Sum of Elements/1, Width/1, MinMax2/1, MinMax3/1
  Width/1 -> Divide/2
  Constant6/1 -> Range_Monotonicity Calculation/1(IDXSELN1_ULS_U08)
  Data Store Read2/1 -> Logical Operator3/1, If1/2
  Data Store Read3/1 -> If1/1, Logical Operator3/2
  Constant7/1 -> Data Store Write2/1, Data Store Write1/1

== system SF007A_SysFricLrng/SysFricLrng/SysFricLrngPer1/RunningAndCalibrationModes/LearningConstraint/VehSpdConstraint ==
  note: Initialize the Temporary Variables
  note: The vehicle speed interval should not overlap.
  note: SysFricLrngVehSpd defines vehicle speed interval limits:
      | the first column defines the low limits, and the second column defines the high limits.
  VehSpd : Inport
  Constant : Constant  Value=false  OutDataTypeStr=boolean
      settings: AttributesFormatString=%<OutDataTypeStr>
  Constant1 : Constant  Value=0  OutDataTypeStr=uint8
      settings: AttributesFormatString=%<OutDataTypeStr>
  Constant2 : Constant  Value=VEHSPDPTNUM1_ULS_U08
  CopyRight2 : Subsystem  Description=|  mask(Copyright Information){none=on}
      | Copyright info block.                                               
      |                                                                     
      | Place copyright information at the top of every subsystem in design.
      mask prompts: none "No parameters"
      mask help: Place copyright information at the top of every subsystem in design.
      mask Display:
      | NxtrConf = 'Nexteer Confidential';
      | 
      | sys = bdroot; %handle for the current model ("system")
      | first = get_param(sys,'Created');
      | first = first(end-3:end);  %year is last four digits
      | 
      | last = get_param(sys,'LastModifiedDate');
      | if isempty(last)
      |     last = datestr(now,'yyyy');
      | else
      |     last = last(end-3:end);
      | end
      | 
      | if strcmp(first,last)
      |     fprintf('%s -- Copyright %s Nexteer',NxtrConf,first)
      | else
      |     fprintf('%s -- %s%s- %s Nexteer',NxtrConf,char(169),first,last)
      | end
  Data Store Memory19 : DataStoreMemory  Description=Local Data Store Memory  DataStoreName=VehSpdIdxTmp_Cnt_T_u08  OutDataTypeStr=uint8
      settings: AttributesFormatString=%<Description>
  Data Store Memory35 : DataStoreMemory  Description=Local Data Store Memory  DataStoreName=VehSpdOkTmp_Cnt_T_lgc  OutDataTypeStr=boolean
      settings: AttributesFormatString=%<Description>
  Data Store Write : DataStoreWrite  Priority=1  DataStoreName=VehSpdOkTmp_Cnt_T_lgc
      settings: AttributesFormatString=Priority:%<Priority>
  Data Store Write1 : DataStoreWrite  Priority=1  DataStoreName=VehSpdIdxTmp_Cnt_T_u08
      settings: AttributesFormatString=Priority:%<Priority>
  VehSpdIdxCalcn : Subsystem  Priority=2  TreatAsAtomicUnit=on
      settings: AttributesFormatString=Priority:%<Priority>
  VehSpdIdx : Outport
  VehSpdOK : Outport  Port=2
  wires:
  VehSpdIdxCalcn/1(VehSpdOK) -> VehSpdOK/1
  VehSpd/1 -> VehSpdIdxCalcn/1(VehSpd)
  Constant/1 -> Data Store Write/1
  Constant1/1 -> Data Store Write1/1
  VehSpdIdxCalcn/2(VehSpdIdx) -> VehSpdIdx/1
  Constant2/1 -> VehSpdIdxCalcn/2(VEHSPDPTNUM1_ULS_U08)

== system SF007A_SysFricLrng/SysFricLrng/SysFricLrngPer1/RunningAndCalibrationModes/PrepData/Column Torque ==
  Ratio : Inport
  HwTq : Inport  Port=2
  MotTqCmdCrf : Inport  Port=3
  CopyRight2 : Subsystem  Description=|  mask(Copyright Information){none=on}
      | Copyright info block.                                               
      |                                                                     
      | Place copyright information at the top of every subsystem in design.
      mask prompts: none "No parameters"
      mask help: Place copyright information at the top of every subsystem in design.
      mask Display:
      | NxtrConf = 'Nexteer Confidential';
      | 
      | sys = bdroot; %handle for the current model ("system")
      | first = get_param(sys,'Created');
      | first = first(end-3:end);  %year is last four digits
      | 
      | last = get_param(sys,'LastModifiedDate');
      | if isempty(last)
      |     last = datestr(now,'yyyy');
      | else
      |     last = last(end-3:end);
      | end
      | 
      | if strcmp(first,last)
      |     fprintf('%s -- Copyright %s Nexteer',NxtrConf,first)
      | else
      |     fprintf('%s -- %s%s- %s Nexteer',NxtrConf,char(169),first,last)
      | end
  Product1 : Product  RndMeth=Zero
  Sum : Sum  Inputs=|++
  ColTq : Outport
  wires:
  MotTqCmdCrf/1 -> Product1/1
  HwTq/1 -> Sum/1
  Ratio/1 -> Product1/2
  Sum/1 -> ColTq/1
  Product1/1 -> Sum/2

== system SF007A_SysFricLrng/SysFricLrng/SysFricLrngPer1/RunningAndCalibrationModes/PrepData/CopyRight2 ==

== system SF007A_SysFricLrng/SysFricLrng/SysFricLrngPer1/RunningAndCalibrationModes/Running Mode/CopyRight2 ==

== system SF007A_SysFricLrng/SysFricLrng/SysFricLrngPer1/RunningAndCalibrationModes/Running Mode/Else Action ==
  In1 : Inport
  Action Port : ActionPort  ActionType=else
  CopyRight2 : Subsystem  Description=|  mask(Copyright Information){none=on}
      | Copyright info block.                                               
      |                                                                     
      | Place copyright information at the top of every subsystem in design.
      mask prompts: none "No parameters"
      mask help: Place copyright information at the top of every subsystem in design.
      mask Display:
      | NxtrConf = 'Nexteer Confidential';
      | 
      | sys = bdroot; %handle for the current model ("system")
      | first = get_param(sys,'Created');
      | if(isempty(first))
      |     first = datestr(now,'yyyy');
      | else
      |     first = first(end-3:end);  %year is last four digits
      | end
      | 
      | last = get_param(sys,'LastModifiedDate');
      | if isempty(last)
      |     last = datestr(now,'yyyy');
      | else
      |     last = last(end-3:end);
      | end
      | 
      | if strcmp(first,last)
      |     fprintf('%s -- Copyright %s Nexteer',NxtrConf,first)
      | else
      |     fprintf('%s -- %s%s- %s Nexteer',NxtrConf,char(169),first,last)
      | end
  Out1 : Outport
  wires:
  In1/1 -> Out1/1

== system SF007A_SysFricLrng/SysFricLrng/SysFricLrngPer1/RunningAndCalibrationModes/Running Mode/If Action Subsystem ==
  VehSpdIdx : Inport
  Action Port : ActionPort  ActionType=then
  BlendingFricChg : Subsystem
  Constant : Constant  Value=SysFricLrngMaskVehSpd
  CopyRight2 : Subsystem  Description=|  mask(Copyright Information){none=on}
      | Copyright info block.                                               
      |                                                                     
      | Place copyright information at the top of every subsystem in design.
      mask prompts: none "No parameters"
      mask help: Place copyright information at the top of every subsystem in design.
      mask Display:
      | NxtrConf = 'Nexteer Confidential';
      | 
      | sys = bdroot; %handle for the current model ("system")
      | first = get_param(sys,'Created');
      | if(isempty(first))
      |     first = datestr(now,'yyyy');
      | else
      |     first = first(end-3:end);  %year is last four digits
      | end
      | 
      | last = get_param(sys,'LastModifiedDate');
      | if isempty(last)
      |     last = datestr(now,'yyyy');
      | else
      |     last = last(end-3:end);
      | end
      | 
      | if strcmp(first,last)
      |     fprintf('%s -- Copyright %s Nexteer',NxtrConf,first)
      | else
      |     fprintf('%s -- %s%s- %s Nexteer',NxtrConf,char(169),first,last)
      | end
  Data Store Read : DataStoreRead  Priority=1  DataStoreName=FricOffs
      settings: AttributesFormatString=Priority=%<Priority>
  Data Store Write : DataStoreWrite  Priority=2  DataStoreName=FricOffs
      settings: AttributesFormatString=Priority=%<Priority>
  If : If  IfExpression=u1
  If Action Subsystem : Subsystem  TreatAsAtomicUnit=on
  Merge : Merge
  Selector3 : Selector  InputPortWidth=4  IndexOptions=Index vector (port)  Indices=[1]  OutputSizes=1
  FricOffs : Outport
  wires:
  Merge/1 -> Data Store Write/1, FricOffs/1
  Constant/1 -> Selector3/1
  VehSpdIdx/1 -> Selector3/2, BlendingFricChg/1(VehSpdIdx)
  Selector3/1 -> If/1
  If/1 -> BlendingFricChg/Action
  BlendingFricChg/1(FilOffs) -> Merge/1
  If/2 -> If Action Subsystem/Action
  If Action Subsystem/1(Out1) -> Merge/2
  Data Store Read/1 -> If Action Subsystem/1(In1)

== system SF007A_SysFricLrng/SysFricLrng/SysFricLrngPer1/UpdateNvmPrm/UpdateVehLearnedFric/CopyRight2 ==

== system SF007A_SysFricLrng/SysFricLrng/SysFricLrngPer1/ResettingMode (reset to baseline) (rename this mode as InitializeTable)/UpdateBaselineFric/InitAvrgFricLpFil1/CopyRight2 ==

== system SF007A_SysFricLrng/SysFricLrng/SysFricLrngPer1/ResettingMode (reset to baseline) (rename this mode as InitializeTable)/UpdateBaselineFric/InitAvrgFricLpFil2/CopyRight2 ==

== system SF007A_SysFricLrng/SysFricLrng/SysFricLrngPer1/ResettingMode (reset to baseline) (rename this mode as InitializeTable)/UpdateBaselineFric/InitAvrgFricLpFil3/CopyRight2 ==

== system SF007A_SysFricLrng/SysFricLrng/SysFricLrngPer1/ResettingMode (reset to baseline) (rename this mode as InitializeTable)/UpdateBaselineFric/InitAvrgFricLpFil4/CopyRight2 ==

== system SF007A_SysFricLrng/SysFricLrng/SysFricLrngPer1/ResettingMode (reset to baseline) (rename this mode as InitializeTable)/UpdateFricLrngHys_RngCntr/Update BaseLine Range Counter/CopyRight2 ==

== system SF007A_SysFricLrng/SysFricLrng/SysFricLrngPer1/ResettingMode (reset to baseline) (rename this mode as InitializeTable)/UpdateFricLrngHys_RngCntr/UpdateFricLrngHys/CopyRight2 ==

== system SF007A_SysFricLrng/SysFricLrng/SysFricLrngPer1/ResettingMode (reset to baseline) (rename this mode as InitializeTable)/UpdateFricLrngHys_RngCntr/UpdateFricLrngHys/Even Rows ==
  note: Don't code this
  note: Add EOLFricDiff to Hys matrix row 2, 4, 6, 8
  HwPtNumIdx : Inport
  VehspdPtNumIdx : Inport  Port=2
  EolFricDif : Inport  Port=3
  Action Port : ActionPort  ActionType=else
  Assignment1 : Assignment  NumberOfDimensions=2  IndexOptions=Index vector (port),Index vector (port)  Indices=1,1  OutputSizes=1,1
  Constant2 : Constant  Value=SysFricLrngBasLineHys
  CopyRight2 : Subsystem  Description=|  mask(Copyright Information){none=on}
      | Copyright info block.                                               
      |                                                                     
      | Place copyright information at the top of every subsystem in design.
      mask prompts: none "No parameters"
      mask help: Place copyright information at the top of every subsystem in design.
      mask Display:
      | NxtrConf = 'Nexteer Confidential';
      | 
      | sys = bdroot; %handle for the current model ("system")
      | first = get_param(sys,'Created');
      | first = first(end-3:end);  %year is last four digits
      | 
      | last = get_param(sys,'LastModifiedDate');
      | if isempty(last)
      |     last = datestr(now,'yyyy');
      | else
      |     last = last(end-3:end);
      | end
      | 
      | if strcmp(first,last)
      |     fprintf('%s -- Copyright %s Nexteer',NxtrConf,first)
      | else
      |     fprintf('%s -- %s%s- %s Nexteer',NxtrConf,char(169),first,last)
      | end
  Data Store Read7 : DataStoreRead  Priority=1  DataStoreName=FricLrngData  DataStoreElements=FricLrngData.Hys(:,:)
      settings: AttributesFormatString=Priority: %<Priority>
  Data Store Write8 : DataStoreWrite  Priority=2  DataStoreName=FricLrngData  DataStoreElements=FricLrngData.Hys(:,:)
      settings: AttributesFormatString=Priority:%<Priority>
  Selector1 : Selector  NumberOfDimensions=2  InputPortWidth=8  IndexOptions=Index vector (port),Index vector (port)  Indices=[1 3],1  OutputSizes=1,1
  Sum1 : Sum  Inputs=|++
  Transpose1 : Math  Operator=transpose  SaturateOnIntegerOverflow=on
  wires:
  Data Store Read7/1 -> Assignment1/1
  Assignment1/1 -> Data Store Write8/1
  Sum1/1 -> Assignment1/2
  Selector1/1 -> Sum1/1
  EolFricDif/1 -> Sum1/2
  Constant2/1 -> Transpose1/1
  HwPtNumIdx/1 -> Assignment1/4, Selector1/3
  VehspdPtNumIdx/1 -> Selector1/2, Assignment1/3
  Transpose1/1 -> Selector1/1

== system SF007A_SysFricLrng/SysFricLrng/SysFricLrngPer1/ResettingMode (reset to baseline) (rename this mode as InitializeTable)/UpdateFricLrngHys_RngCntr/UpdateFricLrngHys/Odd Rows ==
  note: Subtract EOLFricDiff to Hys matrix row 1, 3, 5, 7
  note: Don't code this
  HwPtNumIdx : Inport
  VehspdPtNumIdx : Inport  Port=2
  EolFricDif : Inport  Port=3
  Action Port : ActionPort  ActionType=then
  Assignment1 : Assignment  NumberOfDimensions=2  IndexOptions=Index vector (port),Index vector (port)  Indices=1,1  OutputSizes=1,1
  Constant2 : Constant  Value=SysFricLrngBasLineHys
  CopyRight2 : Subsystem  Description=|  mask(Copyright Information){none=on}
      | Copyright info block.                                               
      |                                                                     
      | Place copyright information at the top of every subsystem in design.
      mask prompts: none "No parameters"
      mask help: Place copyright information at the top of every subsystem in design.
      mask Display:
      | NxtrConf = 'Nexteer Confidential';
      | 
      | sys = bdroot; %handle for the current model ("system")
      | first = get_param(sys,'Created');
      | first = first(end-3:end);  %year is last four digits
      | 
      | last = get_param(sys,'LastModifiedDate');
      | if isempty(last)
      |     last = datestr(now,'yyyy');
      | else
      |     last = last(end-3:end);
      | end
      | 
      | if strcmp(first,last)
      |     fprintf('%s -- Copyright %s Nexteer',NxtrConf,first)
      | else
      |     fprintf('%s -- %s%s- %s Nexteer',NxtrConf,char(169),first,last)
      | end
  Data Store Read7 : DataStoreRead  Priority=1  DataStoreName=FricLrngData  DataStoreElements=FricLrngData.Hys(:,:)
      settings: AttributesFormatString=Priority: %<Priority>
  Data Store Write8 : DataStoreWrite  Priority=2  DataStoreName=FricLrngData  DataStoreElements=FricLrngData.Hys(:,:)
      settings: AttributesFormatString=Priority:%<Priority>
  Selector1 : Selector  NumberOfDimensions=2  InputPortWidth=8  IndexOptions=Index vector (port),Index vector (port)  Indices=[1 3],1  OutputSizes=1,1
  Sum1 : Sum  Inputs=|+-
  Transpose1 : Math  Operator=transpose  SaturateOnIntegerOverflow=on
  wires:
  VehspdPtNumIdx/1 -> Assignment1/3, Selector1/2
  HwPtNumIdx/1 -> Selector1/3, Assignment1/4
  Constant2/1 -> Transpose1/1
  EolFricDif/1 -> Sum1/2
  Selector1/1 -> Sum1/1
  Sum1/1 -> Assignment1/2
  Assignment1/1 -> Data Store Write8/1
  Data Store Read7/1 -> Assignment1/1
  Transpose1/1 -> Selector1/1

== system SF007A_SysFricLrng/SysFricLrng/SysFricLrngPer1/RunningAndCalibrationModes/FricLearning/Calculate Average Friction/CopyRight2 ==

== system SF007A_SysFricLrng/SysFricLrng/SysFricLrngPer1/RunningAndCalibrationModes/FricLearning/Calculate Average Friction/Max Raw Average Calculation ==
  VEHSPDPTNUM1_ULS_U08 : Inport
  CopyRight2 : Subsystem  Description=|  mask(Copyright Information){none=on}
      | Copyright info block.                                               
      |                                                                     
      | Place copyright information at the top of every subsystem in design.
      mask prompts: none "No parameters"
      mask help: Place copyright information at the top of every subsystem in design.
      mask Display:
      | NxtrConf = 'Nexteer Confidential';
      | 
      | sys = bdroot; %handle for the current model ("system")
      | first = get_param(sys,'Created');
      | first = first(end-3:end);  %year is last four digits
      | 
      | last = get_param(sys,'LastModifiedDate');
      | if isempty(last)
      |     last = datestr(now,'yyyy');
      | else
      |     last = last(end-3:end);
      | end
      | 
      | if strcmp(first,last)
      |     fprintf('%s -- Copyright %s Nexteer',NxtrConf,first)
      | else
      |     fprintf('%s -- %s%s- %s Nexteer',NxtrConf,char(169),first,last)
      | end
  Data Store Read1 : DataStoreRead  Priority=1  DataStoreName=MaxRawAvrgFric_HwNwtMtr_T_f32
      settings: AttributesFormatString=Priority: %<Priority>
  Data Store Read3 : DataStoreRead  Priority=1  DataStoreName=RawAvrgFric
      settings: AttributesFormatString=Priority: %<Priority>
  For Iterator : ForIterator  IterationSource=external  IterationVariableDataType=int8
  MaxRawAvrg : Subsystem
  Relational Operator : RelationalOperator  Operator=>  OutDataTypeStr=boolean
  Selector1 : Selector  InputPortWidth=4  IndexOptions=Index vector (port)  Indices=[1 3]  OutputSizes=1
  wires:
  For Iterator/1 -> Selector1/2
  VEHSPDPTNUM1_ULS_U08/1 -> For Iterator/1
  Data Store Read3/1 -> Selector1/1
  Selector1/1 -> MaxRawAvrg/1(MaxRawAvrg), Relational Operator/1
  Data Store Read1/1 -> Relational Operator/2
  Relational Operator/1 -> MaxRawAvrg/Enable
